simulink model "Unit1_ex"  (R2016a)
settings: Solver=ode1  StartTime=0.0  StopTime=0.68  FixedStep=0.02  RelTol=1e-3
InitFcn:
  | m=0.2 % mass in kg
  | g=9.81 % gravity constant
model workspace (MAT data in the model file):
  g = 9.81
  m = 0.2
settings Model: Creator=chris.barlow  LastModifiedBy=chris.barlow

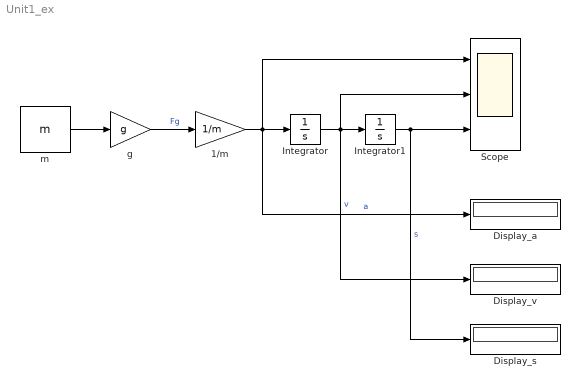
== system Unit1_ex ==
  1/m : Gain  Gain=1/m
  Display_a : Display
  Display_s : Display
  Display_v : Display
  Integrator : Integrator
  Integrator1 : Integrator
      settings: AttributesFormatString=s0 = %<InitialCondition>
  Scope : Scope  NumInputPorts=3
  g : Gain  Gain=g
  m : Constant  Value=m
  wires:
  m/1 -> g/1
  g/1 -> 1/m/1  "Fg"
  1/m/1 -> Scope/1, Display_a/1, Integrator/1  "a"
  Integrator/1 -> Display_v/1, Scope/2, Integrator1/1  "v"
  Integrator1/1 -> Display_s/1, Scope/3  "s"
